simulink model "Troca_marchas"  (R2015a)
settings: Solver=ode45  StartTime=0.0  StopTime=10.0  RelTol=1e-3
settings Model: Creator=PC  LastModifiedBy=PC

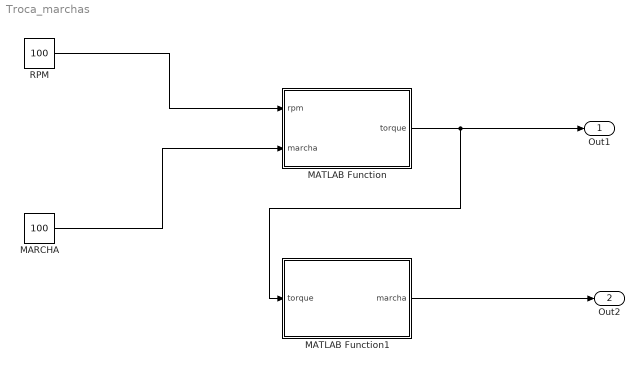
== system Troca_marchas ==
  MARCHA : Constant  Value=100
  MATLAB Function : MATLAB Function  TreatAsAtomicUnit=on
  MATLAB Function1 : MATLAB Function  TreatAsAtomicUnit=on
  RPM : Constant  Value=100
  Out1 : Outport
  Out2 : Outport  Port=2
  wires:
  MATLAB Function/1(torque) -> Out1/1, MATLAB Function1/1(torque)
  MATLAB Function1/1(marcha) -> Out2/1
  RPM/1 -> MATLAB Function/1(rpm)
  MARCHA/1 -> MATLAB Function/2(marcha)

== matlab function Troca_marchas/MATLAB Function1 ==
  data: torque input; marcha output
function marcha = fcn(torque)
    %#codegen

    if torque < 50
        marcha = 0;
    elseif torque >= 350 
        marcha = 1;
    elseif torque >= 300 
        marcha = 2;
    elseif torque >= 250 
        marcha = 3;
    else torque >= 200 
        marcha = 4;
    
    end
end

== matlab function Troca_marchas/MATLAB Function ==
  data: rpm input; torque output; marcha input
function torque = fcn(rpm,marcha)
    %#codegen

    if rpm < 1000 && marcha = 0
        torque = 150;
    elseif rpm >= 1000 && rpm < 2000
        torque = 200;
    elseif rpm >= 2000 && rpm < 3000
        torque = 250;
    elseif rpm >= 3000 && rpm < 4000
        torque = 300;
    else
        torque = 350;
    end
end
